simulink model "Sensor_and_Estimator_Models_with_Star_Tracker"  (R2018b)
settings: Solver=VariableStepAuto  StartTime=0.0  StopTime=10.0  RelTol=1e-3
values from neighbouring files (symbols this model uses):
  noise = 10^-9    (= 1e-09)    [Lab1.m]    (also in Micro_Sat_Open_Loop.m)
  T_e = 0.5    [Lab1.m]    (also in Micro_Sat_Open_Loop.m)
  To_m = 0.8    [Lab1.m]    (also in Micro_Sat_Open_Loop.m)
settings Model: Creator=EKOCULU  LastModifiedBy=EKOCULU

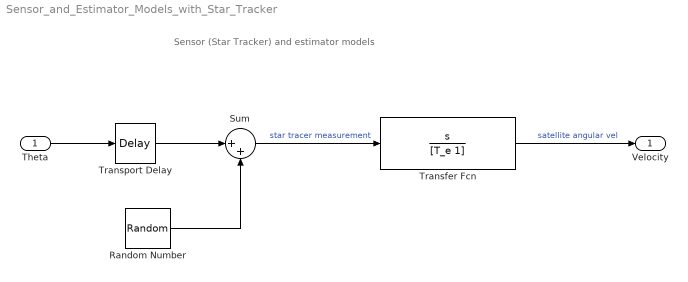
== system Sensor_and_Estimator_Models_with_Star_Tracker ==
  note: Sensor (Star Tracker) and estimator models
  Theta : Inport
  Random Number : RandomNumber  Variance=noise  SampleTime=0.1
  Sum : Sum  Inputs=|++
  Transfer Fcn : TransferFcn  Numerator=[1 0]  Denominator=[T_e 1]
  Transport Delay : TransportDelay  DelayTime=To_m
  Velocity : Outport
  wires:
  Transport Delay/1 -> Sum/1
  Theta/1 -> Transport Delay/1
  Random Number/1 -> Sum/2
  Transfer Fcn/1 -> Velocity/1  "satellite angular vel"
  Sum/1 -> Transfer Fcn/1  "star tracer measurement"
